simulink model "RLproject"  (R2022b)
settings: Solver=ode4  StartTime=0.0  StopTime=Inf  FixedStep=1/500  RelTol=1e-3
model workspace (MAT data in the model file):
  socvcb = containers.Map
  socvcb.serialization.keys = {}
  socvcb.serialization.values = {}
  socvcb.serialization.uniformity = 0
  socvcb.serialization.keyType = 'double'
  socvcb.serialization.valueType = 'any'
undefined symbols (not defined in the file or in its folder): HIL
libraries: quarc_library x10, simulink x4, rllib x1
settings Model: ExtModeTrigDuration=10000  Creator=fvranes  LastModifiedBy=user
settings SolverCC: AlgebraicLoopSolver=TrustRegion
settings DataIOCC: ReturnWorkspaceOutputs=off
settings DebuggingCC: UnderspecifiedInitializationDetection=Classic  MergeDetectMultiDrivingBlocksExec=none  UnconnectedInputMsg=warning  UnconnectedOutputMsg=warning  UnconnectedLineMsg=warning  SFMachineParentedDataDiag=warning
settings ModelReferenceCC: EnableRefExpFcnMdlSchedulingChecks=on  PropagateSignalLabelsOutOfModel=off
settings SFSimCC: CustomCodeUndefinedFunction=UseInterfaceOnly

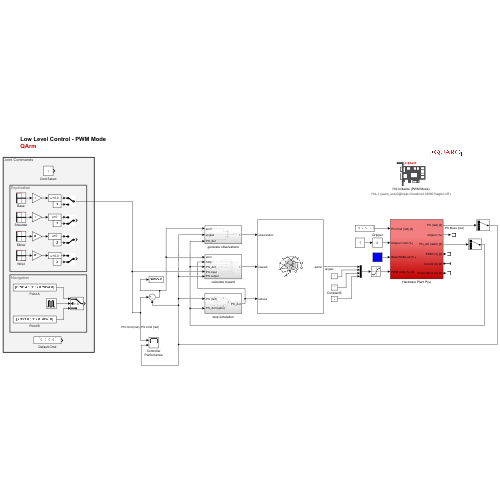
[thumbnail: Simulink's stored preview of the top-level diagram]
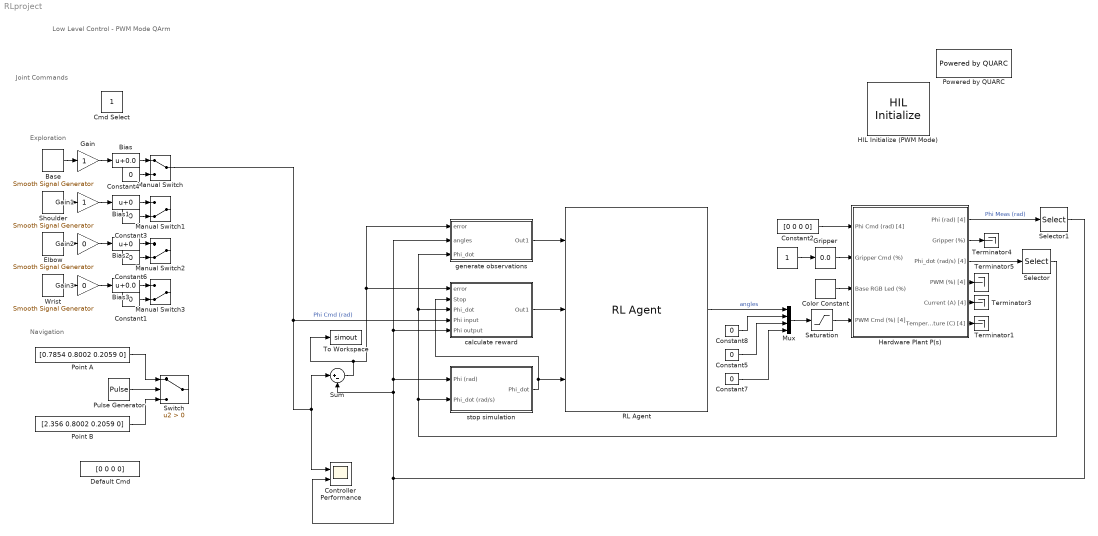
== system RLproject ==
  note: Joint Commands
  note: Exploration
  note: Navigation
  note: Low Level Control - PWM Mode
      | QArm
  " " : Constant
  Base : quarc_library/Sources/Signals/Smooth Signal Generator  signal_type=Square  source=Internal (dialog parameters)  amplitude=pi/4  frequency=0.1  initial_phase=0  sample_time=qc_get_step_size  output_cos=off
      settings: SourceProductName=QUARC Targets
  Bias : Bias  Bias=0.0  SaturateOnIntegerOverflow=off
  Bias1 : Bias  SaturateOnIntegerOverflow=off
  Bias2 : Bias  SaturateOnIntegerOverflow=off
  Bias3 : Bias  Bias=0.0  SaturateOnIntegerOverflow=off
  Cmd Select : Constant
  Color Constant : quarc_library/Sources/Signals/Color Constant  color=[0 0 1]
      settings: SourceProductName=QUARC Targets
  Constant{1,3..8} (7 alike) : Constant  Value=0
  Constant2 : Constant  Value=[0 0 0 0]
  Controller Performance : Scope  NumInputPorts=2
  Default Cmd : Constant  Value=[0 0 0 0]
  Elbow : quarc_library/Sources/Signals/Smooth Signal Generator  signal_type=Square  source=Internal (dialog parameters)  amplitude=pi/4  frequency=0.1  initial_phase=pi  sample_time=qc_get_step_size  output_cos=off
      settings: SourceProductName=QUARC Targets
  Gain : Gain
  Gain1 : Gain
  Gain2 : Gain  Gain=0
  Gain3 : Gain  Gain=0
  Gripper : simulink/Math Operations/Slider Gain  gain=0.0  low=0  high=1
  HIL Initialize (PWM Mode) : quarc_library/Data Acquisition/Generic/Configuration/HIL Initialize  object_name=HIL-1  board_type=qarm_usb  board_number=0@tcpip://localhost:18900?nagle='off'  board_options=j0_mode=1;j1_mode=1;j2_mode=1;j3_mode=1;gripper_mode=0;  exclusive=off  active=on  hardware_clocks=[0]  clock_modes=[]  initial_clock_frequencies=[]  set_clock_params_at_start=off  set_clock_params_at_switch_in=off  set_clock_frequencies_at_start=off  set_clock_frequencies_at_switch_in=off  analog_input_channels=[5:9]  analog_input_configurations=[]  analog_input_maximums=[]  analog_input_minimums=[]  set_analog_input_params_at_start=off  set_analog_input_params_at_switch_in=off  analog_output_channels=[]  analog_output_maximums=inf  analog_output_minimums=-inf  initial_analog_outputs=[0]  final_analog_outputs=[0]  watchdog_analog_outputs=[]  set_analog_output_params_at_start=off  set_analog_output_params_at_switch_in=off  set_analog_outputs_at_start=off  set_analog_outputs_at_switch_in=off  set_analog_outputs_at_terminate=off  set_analog_outputs_at_switch_out=off  set_analog_outputs_on_watchdog=off  digital_input_channels=[]  digital_output_channels=[]  digital_output_configuration=[]  initial_digital_outputs=[0]  final_digital_outputs=[0]  watchdog_digital_outputs=[0]  set_digital_output_params_at_start=off  set_digital_output_params_at_switch_in=off  set_digital_outputs_at_start=off  set_digital_outputs_at_switch_in=off  set_digital_outputs_at_terminate=off  set_digital_outputs_at_switch_out=off  set_digital_outputs_on_watchdog=off  encoder_channels=[]  quadrature=[]  encoder_filter_frequency=[]  initial_encoder_counts=[]  set_encoder_params_at_start=off  set_encoder_params_at_switch_in=off  set_encoder_counts_at_start=off  set_encoder_counts_at_switch_in=off  pwm_channels=[]  pwm_modes=[]  pwm_frequency=[]  pwm_configuration=[]  pwm_alignment=[]  pwm_polarity=[]  pwm_leading_deadband=[]  pwm_trailing_deadband=[]  initial_pwm_outputs=[]  final_pwm_outputs=[]  watchdog_pwm_outputs=[]  set_pwm_params_at_start=off  set_pwm_params_at_switch_in=off  set_pwm_outputs_at_start=off  set_pwm_outputs_at_switch_in=off  set_pwm_outputs_at_terminate=off  set_pwm_outputs_at_switch_out=off  set_pwm_outputs_on_watchdog=off  other_output_channels=[1000:1004 11000:11003 11005:11007]  initial_other_outputs=[zeros(1,9), ones(1,3)]  final_other_outputs=[zeros(1,9), ones(1,3)]  watchdog_other_outputs=zeros(1,12)  set_other_outputs_at_start=off  set_other_outputs_at_switch_in=off  set_other_outputs_at_terminate=on  set_other_outputs_at_switch_out=off  set_other_outputs_on_watchdog=off
  Hardware Plant P(s) : Subsystem
  Manual Switch : ManualSwitch
  Manual Switch1 : ManualSwitch  CurrentSetting=0
  Manual Switch2 : ManualSwitch  CurrentSetting=0
  Manual Switch3 : ManualSwitch  CurrentSetting=0
  Mux : Mux
  Point A : Constant  Value=[0.7854 0.8002 0.2059 0]
  Point B : Constant  Value=[2.356 0.8002 0.2059 0]
  Powered by QUARC : quarc_library/Logos/Powered by QUARC
  Pulse Generator : DiscretePulseGenerator  PulseType=Time based  Period=10  PulseWidth=50
  RL Agent : rllib/RL Agent  Agent=agent_Trained  ExternalActionAsInput=off  ProvideLastAction=off  ProvideCumRwd=off  TreatAsDirectFeedthrough=on  UseStrictObservationDataTypes=off
  Saturation : Saturate  UpperLimit=[1 1 1 1]  LowerLimit=[-1 -1 -1 -1]
  Selector : Selector  InputPortWidth=4  IndexOptions=Index vector (dialog)  Indices=[1]  OutputSizes=1
  Selector1 : Selector  InputPortWidth=4  IndexOptions=Index vector (dialog)  Indices=[1]  OutputSizes=1
  Shoulder : quarc_library/Sources/Signals/Smooth Signal Generator  signal_type=Square  source=Internal (dialog parameters)  amplitude=pi/4  frequency=0.1  initial_phase=0  sample_time=qc_get_step_size  output_cos=off
      settings: SourceProductName=QUARC Targets
  Sum : Sum  Inputs=|+-
  Switch : Switch  Criteria=u2 > Threshold  SaturateOnIntegerOverflow=off  InputSameDT=off
  Terminator{1,3..5} (4 alike) : Terminator
  To Workspace : ToWorkspace  VariableName=simout  SaveFormat=Timeseries  SampleTime=-1
  Wrist : quarc_library/Sources/Signals/Smooth Signal Generator  signal_type=Square  source=Internal (dialog parameters)  amplitude=pi/4  frequency=0.1  initial_phase=0  sample_time=qc_get_step_size  output_cos=off
      settings: SourceProductName=QUARC Targets
  calculate reward : Subsystem
  generate observations : Subsystem
  stop simulation : Subsystem
  wires:
  Color Constant/1 -> Hardware Plant P(s)/3(Base RGB Led (%))
  Hardware Plant P(s)/6(Temperature (C) [4]) -> Terminator1/1
  Hardware Plant P(s)/5(Current (A) [4]) -> Terminator3/1
  Gripper/1 -> Hardware Plant P(s)/2(Gripper Cmd (%))
  Hardware Plant P(s)/2(Gripper (%)) -> Terminator4/1
  Base/1 -> Gain/1
  Shoulder/1 -> Gain1/1
  Constant4/1 -> Manual Switch/2
  Wrist/1 -> Gain3/1
  Constant1/1 -> Manual Switch3/2
  Constant3/1 -> Manual Switch1/2
  Constant6/1 -> Manual Switch2/2
  Manual Switch/1 -> Sum/1, Controller Performance/1, calculate reward/4("Phi input ")  "Phi Cmd (rad)"
  Elbow/1 -> Gain2/1
  " "/1 -> Gripper/1
  Pulse Generator/1 -> Switch/2
  Point B/1 -> Switch/3
  Point A/1 -> Switch/1
  Constant2/1 -> Hardware Plant P(s)/1(Phi Cmd (rad) [4])
  Bias/1 -> Manual Switch/1
  Bias1/1 -> Manual Switch1/1
  Bias2/1 -> Manual Switch2/1
  Bias3/1 -> Manual Switch3/1
  Gain/1 -> Bias/1
  Gain1/1 -> Bias1/1
  Gain2/1 -> Bias2/1
  Gain3/1 -> Bias3/1
  generate observations/1(Out1) -> RL Agent/1
  Sum/1 -> To Workspace/1, generate observations/1(error), calculate reward/1("error  ")
  calculate reward/1(Out1) -> RL Agent/2
  stop simulation/1(Phi_dot) -> calculate reward/2("Stop "), RL Agent/3
  Hardware Plant P(s)/1(Phi (rad) [4]) -> Selector1/1  "Phi Meas (rad)"
  Hardware Plant P(s)/3(Phi_dot (rad/s) [4]) -> Selector/1
  Selector1/1 -> generate observations/2(angles), calculate reward/5(Phi output), stop simulation/1("Phi (rad) "), Sum/2, Controller Performance/2
  Constant8/1 -> Mux/2
  Constant5/1 -> Mux/3
  Constant7/1 -> Mux/4
  Selector/1 -> generate observations/3(Phi_dot), calculate reward/3(Phi_dot), stop simulation/2("Phi_dot (rad/s) ")
  Saturation/1 -> Hardware Plant P(s)/4(PWM Cmd (%) [4])
  Mux/1 -> Saturation/1
  RL Agent/1 -> Mux/1  "angles"
  Hardware Plant P(s)/4(PWM (%) [4]) -> Terminator5/1

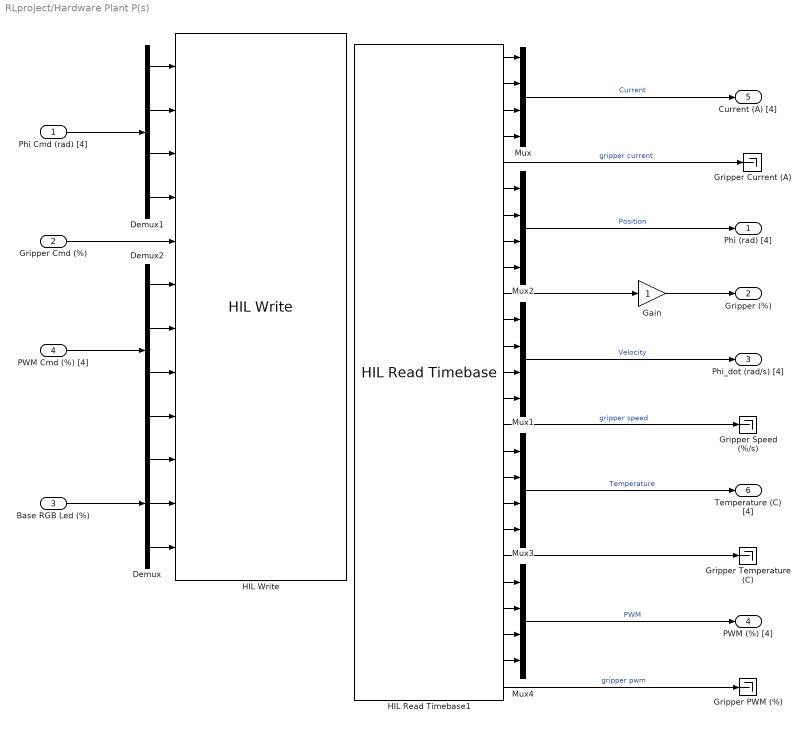
== system RLproject/Hardware Plant P(s) ==
  Phi Cmd (rad) [4] : Inport
  Gripper Cmd (%) : Inport  Port=2
  Base RGB Led (%) : Inport  Port=3
  PWM Cmd (%) [4] : Inport  Port=4
  Demux : Demux  Outputs=3
  Demux1 : Demux
  Demux2 : Demux
  Gain : Gain
  Gripper Current (A) : Terminator
  Gripper PWM (%) : Terminator
  Gripper Speed (%/s) : Terminator
  Gripper Temperature (C) : Terminator
  HIL Read Timebase1 : quarc_library/Data Acquisition/Generic/Timebases/HIL Read Timebase  object_name=HIL-1  clock=0  analog_channels=[5:9]  encoder_channels=[]  digital_channels=[]  other_channels=[1000:1004 3000:3004 10000:10004 11000:11004]  active=on  vector_output=off  data_type_mode=Inherit via back propagation  encoder_data_type=double  digital_data_type=boolean  overflow_mode=Synchronize (for simulated cards only)  samples_in_buffer=1
  HIL Write : quarc_library/Data Acquisition/Generic/Immediate I//O/HIL Write  object_name=HIL-1  analog_channels=[]  pwm_channels=[]  digital_channels=[]  other_channels=[1000:1004 11000:11003 11005:11007]  sample_time=-1  active=on  vector_input=off
  Mux{,1..4} (5 alike) : Mux
  Phi (rad) [4] : Outport  VectorParamsAs1DForOutWhenUnconnected=off
  Gripper (%) : Outport  Port=2  VectorParamsAs1DForOutWhenUnconnected=off
  Phi_dot (rad/s) [4] : Outport  Port=3  VectorParamsAs1DForOutWhenUnconnected=off
  PWM (%) [4] : Outport  Port=4  VectorParamsAs1DForOutWhenUnconnected=off
  Current (A) [4] : Outport  Port=5  VectorParamsAs1DForOutWhenUnconnected=off
  Temperature (C) [4] : Outport  Port=6  VectorParamsAs1DForOutWhenUnconnected=off
  wires:
  HIL Read Timebase1/14 -> Mux1/4
  HIL Read Timebase1/9 -> Mux2/4
  HIL Read Timebase1/6 -> Mux2/1
  HIL Read Timebase1/18 -> Mux3/3
  HIL Read Timebase1/8 -> Mux2/3
  HIL Read Timebase1/12 -> Mux1/2
  HIL Read Timebase1/4 -> Mux/4
  HIL Read Timebase1/7 -> Mux2/2
  HIL Read Timebase1/5 -> Gripper Current (A)/1  "gripper current"
  HIL Read Timebase1/15 -> Gripper Speed (%/s)/1  "gripper speed"
  Demux/3 -> HIL Write/12
  HIL Read Timebase1/3 -> Mux/3
  HIL Read Timebase1/17 -> Mux3/2
  HIL Read Timebase1/16 -> Mux3/1
  HIL Read Timebase1/11 -> Mux1/1
  Demux/1 -> HIL Write/10
  HIL Read Timebase1/19 -> Mux3/4
  Demux/2 -> HIL Write/11
  HIL Read Timebase1/13 -> Mux1/3
  HIL Read Timebase1/2 -> Mux/2
  HIL Read Timebase1/1 -> Mux/1
  HIL Read Timebase1/20 -> Gripper Temperature (C)/1
  Mux/1 -> Current (A) [4]/1  "Current"
  Mux1/1 -> Phi_dot (rad/s) [4]/1  "Velocity"
  Mux3/1 -> Temperature (C) [4]/1  "Temperature"
  Base RGB Led (%)/1 -> Demux/1
  Demux1/1 -> HIL Write/1
  Demux1/2 -> HIL Write/2
  Demux1/3 -> HIL Write/3
  Demux1/4 -> HIL Write/4
  Phi Cmd (rad) [4]/1 -> Demux1/1
  PWM Cmd (%) [4]/1 -> Demux2/1
  Demux2/1 -> HIL Write/6
  Demux2/2 -> HIL Write/7
  Demux2/3 -> HIL Write/8
  Demux2/4 -> HIL Write/9
  Mux2/1 -> Phi (rad) [4]/1  "Position"
  HIL Read Timebase1/21 -> Mux4/1
  HIL Read Timebase1/22 -> Mux4/2
  HIL Read Timebase1/23 -> Mux4/3
  HIL Read Timebase1/24 -> Mux4/4
  HIL Read Timebase1/25 -> Gripper PWM (%)/1  "gripper pwm"
  Mux4/1 -> PWM (%) [4]/1  "PWM"
  HIL Read Timebase1/10 -> Gain/1
  Gain/1 -> Gripper (%)/1
  Gripper Cmd (%)/1 -> HIL Write/5

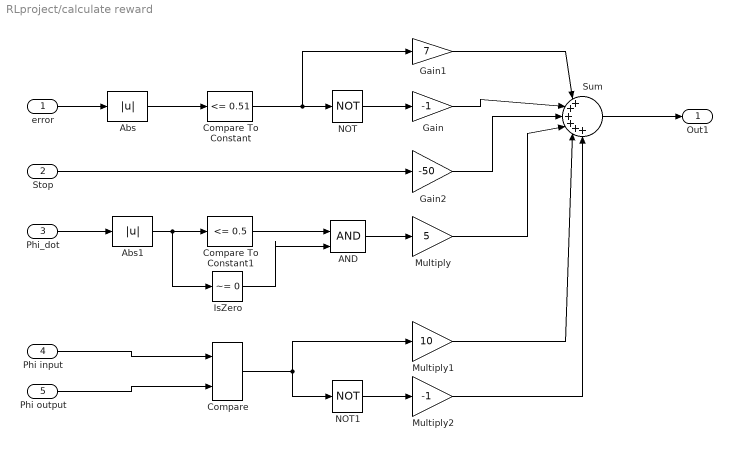
== system RLproject/calculate reward ==
  "error  " : Inport
  "Stop " : Inport  Port=2
  Phi_dot : Inport  Port=3
  "Phi input " : Inport  Port=4
  Phi output : Inport  Port=5
  AND : Logic  IconShape=distinctive  AllPortsSameDT=off  OutDataTypeStr=boolean
  Abs : Abs  SaturateOnIntegerOverflow=off
  Abs1 : Abs  SaturateOnIntegerOverflow=off
  Compare : quarc_library/Logic Operations/Compare  operator===  output_data_type=boolean
      settings: SourceProductName=QUARC Targets
  Compare To Constant : simulink/Logic and Bit Operations/Compare To Constant  relop=<=  const=0.51  OutDataTypeStr=boolean
  Compare To Constant1 : simulink/Logic and Bit Operations/Compare To Constant  relop=<=  const=0.5  OutDataTypeStr=boolean
  Gain : Gain  Gain=-1
  Gain1 : Gain  Gain=7
  Gain2 : Gain  Gain=-50
  IsZero : simulink/Logic and Bit Operations/Compare To Zero  relop=~=  OutDataTypeStr=boolean
      settings: LibrarySourceBlock=|
      | simulink/Quick Insert/Logic and Bit
      | Operations/IsZero
  Multiply : Gain  Gain=5
  Multiply1 : Gain  Gain=10
  Multiply2 : Gain  Gain=-1
  NOT : Logic  Operator=NOT  IconShape=distinctive  AllPortsSameDT=off  OutDataTypeStr=boolean
  NOT1 : Logic  Operator=NOT  IconShape=distinctive  AllPortsSameDT=off  OutDataTypeStr=boolean
  Sum : Sum  Inputs=|++++++
  Out1 : Outport
  wires:
  "error  "/1 -> Abs/1
  Compare To Constant/1 -> Gain1/1, NOT/1
  NOT/1 -> Gain/1
  "Stop "/1 -> Gain2/1
  Sum/1 -> Out1/1
  Abs/1 -> Compare To Constant/1
  Gain1/1 -> Sum/1
  Gain/1 -> Sum/2
  Gain2/1 -> Sum/3
  Abs1/1 -> IsZero/1, Compare To Constant1/1
  Phi_dot/1 -> Abs1/1
  IsZero/1 -> AND/2
  Compare To Constant1/1 -> AND/1
  AND/1 -> Multiply/1
  "Phi input "/1 -> Compare/1
  Phi output/1 -> Compare/2
  Compare/1 -> Multiply1/1, NOT1/1
  NOT1/1 -> Multiply2/1
  Multiply/1 -> Sum/4
  Multiply1/1 -> Sum/5
  Multiply2/1 -> Sum/6

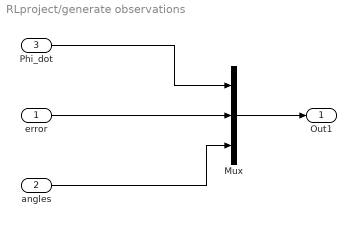
== system RLproject/generate observations ==
  error : Inport
  angles : Inport  Port=2
  Phi_dot : Inport  Port=3
  Mux : Mux  Inputs=3
  Out1 : Outport
  wires:
  Mux/1 -> Out1/1
  Phi_dot/1 -> Mux/1
  error/1 -> Mux/2
  angles/1 -> Mux/3

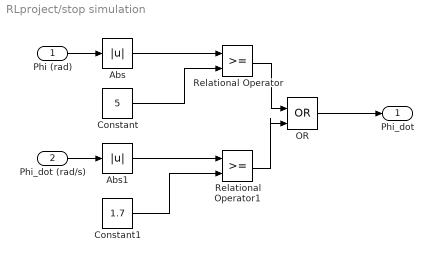
== system RLproject/stop simulation ==
  "Phi (rad) " : Inport
  "Phi_dot (rad/s) " : Inport  Port=2
  Abs : Abs  SaturateOnIntegerOverflow=off
  Abs1 : Abs  SaturateOnIntegerOverflow=off
  Constant : Constant  Value=5
  Constant1 : Constant  Value=1.7
  OR : Logic  Operator=OR  IconShape=distinctive  AllPortsSameDT=off  OutDataTypeStr=boolean
  Relational Operator : RelationalOperator  OutDataTypeStr=boolean  RndMeth=Simplest  InputSameDT=off
  Relational Operator1 : RelationalOperator  OutDataTypeStr=boolean  RndMeth=Simplest  InputSameDT=off
  Phi_dot : Outport
  wires:
  "Phi (rad) "/1 -> Abs/1
  Constant/1 -> Relational Operator/2
  Abs/1 -> Relational Operator/1
  "Phi_dot (rad/s) "/1 -> Abs1/1
  Abs1/1 -> Relational Operator1/1
  Constant1/1 -> Relational Operator1/2
  Relational Operator/1 -> OR/1
  Relational Operator1/1 -> OR/2
  OR/1 -> Phi_dot/1
